simulink model "reflinear"  (Simulink 2.20)
settings: Solver=ode45  StartTime=0.0  StopTime=10  RelTol=1e-3  AbsTol=1e-6
values from neighbouring files (symbols this model uses):
  kdc = dcgain(clsystem)    [leadreg.m]    (also in reference.m)
undefined symbols (not defined in the file or in its folder): denr, numr
libraries: simulink_extras x3
settings Model: ConsistencyChecking=off  RTWPlaceOutputsASAP=off

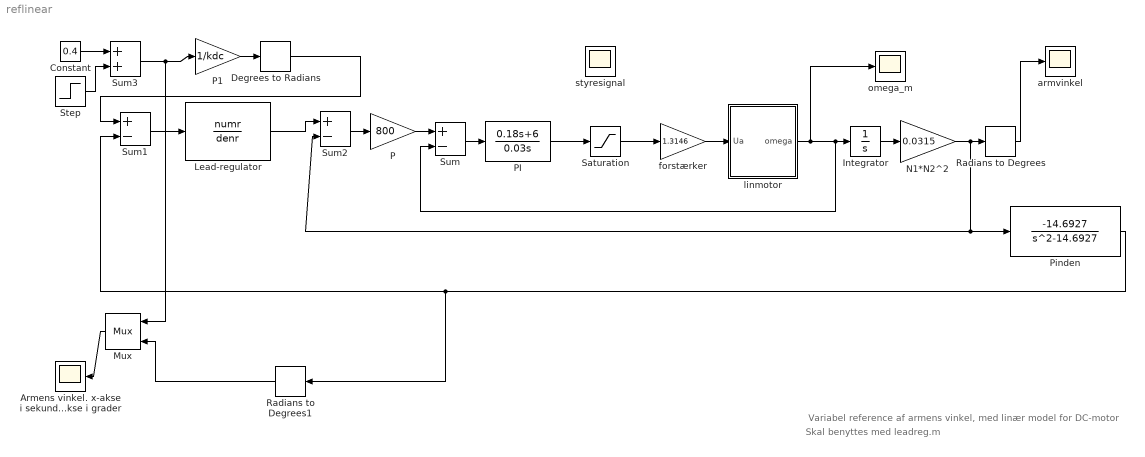
== system reflinear ==
  note: Variabel reference af armens vinkel, med linær model for DC-motor
  note: Skal benyttes med leadreg.m
  Armens vinkel. x-akse i sekunder og y-akse i grader : Scope
      settings: TickLabels=on  TimeRange=5  YMin=-1  YMax=1  SaveToWorkspace=off  SaveName=ScopeData
  Constant : Constant  Value=0.4
  Degrees to Radians : simulink_extras/Transformations/Degrees to Radians
  Integrator : Integrator  ExternalReset=none  InitialConditionSource=internal  InitialCondition=0  LimitOutput=off  UpperSaturationLimit=inf  LowerSaturationLimit=-inf  ShowSaturationPort=off  ShowStatePort=off  AbsoluteTolerance=auto
  Lead-regulator : TransferFcn  Numerator=numr  Denominator=denr
  Mux : Mux  Orientation=left  Inputs=2
  N1*N2^2 : Gain  Gain=0.0315
  P : Gain  Gain=800
  P1 : Gain  Gain=1/kdc
  PI : TransferFcn  Numerator=[0.18 6]  Denominator=[0.03 0]
  Pinden : TransferFcn  Numerator=[-14.6927]  Denominator=[1 0 -14.6927 ]
  Radians to Degrees : simulink_extras/Transformations/Radians to Degrees
  Radians to Degrees1 : simulink_extras/Transformations/Radians to Degrees  Orientation=left
  Saturation : Saturate  UpperLimit=5  LowerLimit=-5
  Step : Step  Time=5  Before=0  After=-0.7
  Sum : Sum  Inputs=+-
  Sum1 : Sum  Inputs=+-
  Sum2 : Sum  Inputs=+-
  Sum3 : Sum  Inputs=++
  armvinkel : Scope
      settings: TickLabels=on  TimeRange=10  YMin=-0.00065  YMax=0  SaveToWorkspace=off  SaveName=ScopeData
  forstærker : Gain  Gain=1.3146
  linmotor : Subsystem
  "omega_m " : Scope
      settings: TickLabels=on  TimeRange=10  YMin=-0.00065  YMax=0  SaveToWorkspace=off  SaveName=ScopeData
  styresignal : Scope
      settings: TickLabels=on  TimeRange=0.5  YMin=0  YMax=13  SaveToWorkspace=off  SaveName=ScopeData
  wires:
  Sum/1 -> PI/1
  Saturation/1 -> forstærker/1
  Integrator/1 -> N1*N2^2/1
  Radians to Degrees/1 -> armvinkel/1
  PI/1 -> Saturation/1
  N1*N2^2/1 -> Radians to Degrees/1, Pinden/1, Sum2/2
  P/1 -> Sum/1
  Sum2/1 -> P/1
  Degrees to Radians/1 -> Sum1/1
  Lead-regulator/1 -> Sum2/1
  Pinden/1 -> Sum1/2, Radians to Degrees1/1
  Sum1/1 -> Lead-regulator/1
  P1/1 -> Degrees to Radians/1
  Step/1 -> Sum3/2
  Constant/1 -> Sum3/1
  Sum3/1 -> P1/1, Mux/1
  Radians to Degrees1/1 -> Mux/2
  Mux/1 -> Armens vinkel. x-akse i sekunder og y-akse i grader/1
  linmotor/1(omega) -> Integrator/1, Sum/2, "omega_m "/1
  forstærker/1 -> linmotor/1(Ua)

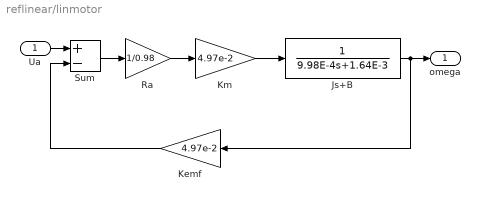
== system reflinear/linmotor ==
  Ua : Inport  Port=1  PortWidth=-1  SampleTime=-1
  Js+B : TransferFcn  Numerator=[1]  Denominator=[9.98E-4 1.64E-3]
  Kemf : Gain  Orientation=left  Gain=4.97e-2
  Km : Gain  Gain=4.97e-2
  Ra : Gain  Gain=1/0.98
  Sum : Sum  Inputs=+-
  omega : Outport  Port=1  InitialOutput=0
  wires:
  Ra/1 -> Km/1
  Sum/1 -> Ra/1
  Kemf/1 -> Sum/2
  Js+B/1 -> Kemf/1, omega/1
  Ua/1 -> Sum/1
  Km/1 -> Js+B/1
